simulink library "Simple_lib"  (R2018b)
settings: Solver=ode45  StartTime=0.0  StopTime=10.0  RelTol=1e-3  EnableMultiTasking=on
undefined symbols (not defined in the file or in its folder): Acceptance, beta, C, C_J, C_P, c_wall, dGain, DiscIntNeverNeededParam, Duplex, Electrical_lib, grab, h_fe, i, i3, K_T, Kman, KmanCE, mu_s, n_rev, R_arm, Simplex, systemTs, tau_0, TinIC, Ts, w_0, wallMass, Watch_lib
libraries: $bdroot x407, PlantUtilityBlockset_lib x30, peGeneralControl x22, simulink x11
(part 7 of 14)

== system Simple_lib/Electrical/Thyristor ==
  In1 : Inport
  c : Inport  Port=2
  In2 : Inport  Port=3
  1/R1 : Gain  Gain=-1
  1/R2 : Gain  Gain=-1
  Discrete-Time Integrator1 : DiscreteIntegrator  gainval=1/10/Ts  SampleTime=Ts  ICPrevOutput=DiscIntNeverNeededParam  ICPrevScaledInput=DiscIntNeverNeededParam
  Saturation : Saturate  UpperLimit=Inf  LowerLimit=0
  Simplex : $bdroot/Utility/Push  Tag=Electrical  SystemSampleTime=-1
  Simplex1 : $bdroot/Utility/Push  Tag=Electrical  SystemSampleTime=-1
  Sum : Sum  Inputs=+|+
  Sum1 : Sum  Inputs=|+-
  conductance : Product
  wires:
  Saturation/1 -> Sum1/1
  conductance/1 -> Saturation/1
  In1/1 -> Simplex/1
  Simplex/1 -> 1/R2/1
  1/R2/1 -> Sum/1
  Sum/1 -> conductance/2
  In2/1 -> Simplex1/1
  Simplex1/1 -> Sum/2
  1/R1/1 -> Simplex1/2
  Sum1/1 -> Discrete-Time Integrator1/1
  Discrete-Time Integrator1/1 -> Simplex/2, 1/R1/1, Sum1/2
  c/1 -> conductance/1

== system Simple_lib/Electrical/Tran ==
  In1 : Inport
  gain : Inport  Port=2
  Duplex : $bdroot/Utility/Output  Tag=Electrical  Level=Level  Flow=flow
  Multiply : Product
  Multiply1 : Product
  Simplex : $bdroot/Utility/Input  Tag=Electrical  Level=V  Flow=I
  Sum1 : Sum  Inputs=+
  Out1 : Outport
  wires:
  Duplex/2 -> Sum1/1
  Duplex/1 -> Out1/1
  Simplex/1 -> Multiply/1
  In1/1 -> Simplex/1
  Multiply1/1 -> Simplex/2
  Multiply/1 -> Duplex/1
  Sum1/1 -> Multiply1/2
  gain/1 -> Multiply1/1, Multiply/2

== system Simple_lib/Electrical/V ==
  C : PlantUtilityBlockset_lib/Electrical/C  C=.1
  Ground : Ground
  Out1 : Outport
  wires:
  C/1 -> Out1/1
  Ground/1 -> C/1

== system Simple_lib/Electrical/VM ==
  note: Does not need duplex
  In1 : Inport
  In2 : Inport  Port=2
  1/R2 : Gain  Gain=-1
  Sum : Sum  Inputs=+|+
  Out1 : Outport
  wires:
  In2/1 -> 1/R2/1
  Sum/1 -> Out1/1
  In1/1 -> Sum/1
  1/R2/1 -> Sum/2

== system Simple_lib/Electrical/VR ==
  In1 : Inport
  R : Inport  Port=2
  Bus Creator : BusCreator  Inputs=2
  Bus Selector : BusSelector  OutputSignals=V,R
  Inflow : $bdroot/Utility/Inflow  SystemSampleTime=-1
  Multiply : Product
  Outflow : $bdroot/Utility/Outflow  Tag=Electrical  SystemSampleTime=-1
  Sum2 : Sum  Inputs=|++
  Sum3 : Sum  Inputs=|+-
  Sum4 : Sum  Inputs=+  CollapseMode=Specified dimension  CollapseDim=2
  Out1 : Outport
  wires:
  Outflow/1 -> Out1/1
  Bus Creator/1 -> Outflow/1
  Sum3/1 -> Bus Creator/1  "V"
  Sum4/1 -> Inflow/2, Multiply/2  "I"
  Bus Selector/1 -> Sum3/1  "<V>"
  Multiply/1 -> Sum3/2
  Outflow/2 -> Sum4/1
  Inflow/1 -> Bus Selector/1
  R/1 -> Multiply/1, Sum2/2
  Sum2/1 -> Bus Creator/2  "R"
  In1/1 -> Inflow/1
  Bus Selector/2 -> Sum2/1  "<R>"

== system Simple_lib/Electrical/VS ==
  In2 : Inport
  Duplex : PlantUtilityBlockset_lib/Utility/Pull  Tag=Electrical  SystemSampleTime=-1
  Terminator : Terminator
  Out1 : Outport
  wires:
  In2/1 -> Duplex/1
  Duplex/2 -> Terminator/1
  Duplex/1 -> Out1/1

== system Simple_lib/Electrical/VStep ==
  In2 : Inport
  Duplex : PlantUtilityBlockset_lib/Utility/Pull  Tag=Electrical  SystemSampleTime=-1
  Terminator : Terminator
  Out1 : Outport
  wires:
  Duplex/1 -> Out1/1
  Duplex/2 -> Terminator/1
  In2/1 -> Duplex/1

== system Simple_lib/Electrical/Windings ==
  Eabc : Inport
  A : Inport  Port=2
  B : Inport  Port=3
  C : Inport  Port=4
  Demux : Demux  Outputs=3
  IM : Subsystem  AncestorBlock=PlantUtilityBlockset_lib/Electrical/IM  mask{R=1}
      mask prompts: R "Resistance"
      mask Display:
      | color('white')
      | plot([-1 1 1 -1 -1], [-1 -1 1 1 -1])
      | color('black')
      | plot([1.0 1.18 1.18 1.0], [0 .2 -.2 0]+.4)
      | plot([-1 -.9 -.5 0 .5 .9 1  .9  .5  0 -.5 -.9 -1],      [ 0  .5 .9 1 .9 .5 0 -.5 -.9 -1 -.9 -.5  0]);
      | text(0,0, 'A')
  IM1 : Subsystem  AncestorBlock=PlantUtilityBlockset_lib/Electrical/IM  mask{R=1}
      mask prompts: R "Resistance"
      mask Display:
      | color('white')
      | plot([-1 1 1 -1 -1], [-1 -1 1 1 -1])
      | color('black')
      | plot([1.0 1.18 1.18 1.0], [0 .2 -.2 0]+.4)
      | plot([-1 -.9 -.5 0 .5 .9 1  .9  .5  0 -.5 -.9 -1],      [ 0  .5 .9 1 .9 .5 0 -.5 -.9 -1 -.9 -.5  0]);
      | text(0,0, 'A')
  IM2 : Subsystem  AncestorBlock=PlantUtilityBlockset_lib/Electrical/IM  mask{R=1}
      mask prompts: R "Resistance"
      mask Display:
      | color('white')
      | plot([-1 1 1 -1 -1], [-1 -1 1 1 -1])
      | color('black')
      | plot([1.0 1.18 1.18 1.0], [0 .2 -.2 0]+.4)
      | plot([-1 -.9 -.5 0 .5 .9 1  .9  .5  0 -.5 -.9 -1],      [ 0  .5 .9 1 .9 .5 0 -.5 -.9 -1 -.9 -.5  0]);
      | text(0,0, 'A')
  L1 : Subsystem  AncestorBlock=PlantUtilityBlockset_lib/Electrical/L1  mask{L=1}
      mask prompts: L "Inductance"
      mask Display:
      | %color('black')
      | plot(   [    0     0.3827     0.7071     0.9239     1.0000     0.9239     0.7071     0.3827     0.0000    -0.3827    -0.7071    -0.9239    -1.0000    -0.9239    -0.7071    -0.3827    -0.0000     0.3827     0.7071     0.9239     1.0000     0.9239     0.7071     0.3827     0.0000    -0.3827    -0.7071    -0.9239    -1.0000    -0.9239    -0.7071    -0.3827    -0.0000     0.3827     0.7071     0.9239     1.0000     0.9239     0.7071     0.3827     0.0000    -0.3827    -0.7071    -0.9239    -1.0000    -0.9239    -0.7071    -0.3827    -0.0000     0.3827     0.7071     0.9239     1.0000     0.9239     0.7071     0.3827     0.0000    -0.3827    -0.7071    -0.9239    -1.0000    -0.9239    -0.7071    -0.3827    -0.0000],   -.5+[-0.0625    -0.0421    -0.0129     0.0230     0.0625     0.1020     0.1379     0.1671     0.1875     0.1984     0.2004     0.1958     0.1875     0.1792     0.1746     0.1766     0.1875     0.2079     0.2371     0.2730     0.3125     0.3520     0.3879     0.4171     0.4375     0.4484     0.4504     0.4458     0.4375     0.4292     0.4246     0.4266     0.4375     0.4579     0.4871     0.5230     0.5625     0.6020     0.6379     0.6671     0.6875     0.6984     0.7004     0.6958     0.6875     0.6792     0.6746     0.6766     0.6875     0.7079     0.7371     0.7730     0.8125     0.8520     0.8879     0.9171     0.9375     0.9484     0.9504     0.9458     0.9375     0.9292     0.9246     0.9266     0.9375])
      | color('white')
      | plot([-1 1 1 -1 -1], [-1 -1 1 1 -1])
  L2 : Subsystem  AncestorBlock=PlantUtilityBlockset_lib/Electrical/L1  mask{L=1}
      mask prompts: L "Inductance"
      mask Display:
      | %color('black')
      | plot(   [    0     0.3827     0.7071     0.9239     1.0000     0.9239     0.7071     0.3827     0.0000    -0.3827    -0.7071    -0.9239    -1.0000    -0.9239    -0.7071    -0.3827    -0.0000     0.3827     0.7071     0.9239     1.0000     0.9239     0.7071     0.3827     0.0000    -0.3827    -0.7071    -0.9239    -1.0000    -0.9239    -0.7071    -0.3827    -0.0000     0.3827     0.7071     0.9239     1.0000     0.9239     0.7071     0.3827     0.0000    -0.3827    -0.7071    -0.9239    -1.0000    -0.9239    -0.7071    -0.3827    -0.0000     0.3827     0.7071     0.9239     1.0000     0.9239     0.7071     0.3827     0.0000    -0.3827    -0.7071    -0.9239    -1.0000    -0.9239    -0.7071    -0.3827    -0.0000],   -.5+[-0.0625    -0.0421    -0.0129     0.0230     0.0625     0.1020     0.1379     0.1671     0.1875     0.1984     0.2004     0.1958     0.1875     0.1792     0.1746     0.1766     0.1875     0.2079     0.2371     0.2730     0.3125     0.3520     0.3879     0.4171     0.4375     0.4484     0.4504     0.4458     0.4375     0.4292     0.4246     0.4266     0.4375     0.4579     0.4871     0.5230     0.5625     0.6020     0.6379     0.6671     0.6875     0.6984     0.7004     0.6958     0.6875     0.6792     0.6746     0.6766     0.6875     0.7079     0.7371     0.7730     0.8125     0.8520     0.8879     0.9171     0.9375     0.9484     0.9504     0.9458     0.9375     0.9292     0.9246     0.9266     0.9375])
      | color('white')
      | plot([-1 1 1 -1 -1], [-1 -1 1 1 -1])
  L3 : Subsystem  AncestorBlock=PlantUtilityBlockset_lib/Electrical/L1  mask{L=1}
      mask prompts: L "Inductance"
      mask Display:
      | %color('black')
      | plot(   [    0     0.3827     0.7071     0.9239     1.0000     0.9239     0.7071     0.3827     0.0000    -0.3827    -0.7071    -0.9239    -1.0000    -0.9239    -0.7071    -0.3827    -0.0000     0.3827     0.7071     0.9239     1.0000     0.9239     0.7071     0.3827     0.0000    -0.3827    -0.7071    -0.9239    -1.0000    -0.9239    -0.7071    -0.3827    -0.0000     0.3827     0.7071     0.9239     1.0000     0.9239     0.7071     0.3827     0.0000    -0.3827    -0.7071    -0.9239    -1.0000    -0.9239    -0.7071    -0.3827    -0.0000     0.3827     0.7071     0.9239     1.0000     0.9239     0.7071     0.3827     0.0000    -0.3827    -0.7071    -0.9239    -1.0000    -0.9239    -0.7071    -0.3827    -0.0000],   -.5+[-0.0625    -0.0421    -0.0129     0.0230     0.0625     0.1020     0.1379     0.1671     0.1875     0.1984     0.2004     0.1958     0.1875     0.1792     0.1746     0.1766     0.1875     0.2079     0.2371     0.2730     0.3125     0.3520     0.3879     0.4171     0.4375     0.4484     0.4504     0.4458     0.4375     0.4292     0.4246     0.4266     0.4375     0.4579     0.4871     0.5230     0.5625     0.6020     0.6379     0.6671     0.6875     0.6984     0.7004     0.6958     0.6875     0.6792     0.6746     0.6766     0.6875     0.7079     0.7371     0.7730     0.8125     0.8520     0.8879     0.9171     0.9375     0.9484     0.9504     0.9458     0.9375     0.9292     0.9246     0.9266     0.9375])
      | color('white')
      | plot([-1 1 1 -1 -1], [-1 -1 1 1 -1])
  Mux : Mux  Inputs=3
  R : Subsystem  AncestorBlock=PlantUtilityBlockset_lib/Electrical/R  mask{R=1}
      mask prompts: R "Resistance"
      mask Display:
      | color('white')
      | plot([-1 1 1 -1 -1], [-1 -1 1 1 -1])
      | color('black')
      | plot([1.0 1.18 1.18 1.0], [0 .2 -.2 0])
      | plot([-8:8]/8, [0 1 0 -1 0 1 0 -1 0 1 0 -1 0 1 0 -1 0])
  R1 : Subsystem  AncestorBlock=PlantUtilityBlockset_lib/Electrical/R  mask{R=1}
      mask prompts: R "Resistance"
      mask Display:
      | color('white')
      | plot([-1 1 1 -1 -1], [-1 -1 1 1 -1])
      | color('black')
      | plot([1.0 1.18 1.18 1.0], [0 .2 -.2 0])
      | plot([-8:8]/8, [0 1 0 -1 0 1 0 -1 0 1 0 -1 0 1 0 -1 0])
  R2 : Subsystem  AncestorBlock=PlantUtilityBlockset_lib/Electrical/R  mask{R=1}
      mask prompts: R "Resistance"
      mask Display:
      | color('white')
      | plot([-1 1 1 -1 -1], [-1 -1 1 1 -1])
      | color('black')
      | plot([1.0 1.18 1.18 1.0], [0 .2 -.2 0])
      | plot([-8:8]/8, [0 1 0 -1 0 1 0 -1 0 1 0 -1 0 1 0 -1 0])
  Terminator : Terminator
  Terminator1 : Terminator
  Terminator2 : Terminator
  Va : Subsystem  Tag=Electrical  AncestorBlock=PlantUtilityBlockset_lib/Utility/Pull  InitFcn=initDuplex
      mask Display:
      | color('white')
      | plot([0 3], [2 2])
      | plot([0 3], [-2 -2])
      | color('black')
      | 
      | plot([0 1 1], [0 0 0.4])
      | plot([1 1 3], [0.6 1 1])
      | plot([1 3 2 1 0 2], [0.6 0.6 0.4 0.6 0.4 0.4])
      | patch([0 2 1],[0.4 0.4 0.6],[0,0,0])
      | plot([3 2 2], [1 1 0.6])
      | plot([2 2 3], [0.4 -1 -1])
  Vb : Subsystem  Tag=Electrical  AncestorBlock=PlantUtilityBlockset_lib/Utility/Pull  InitFcn=initDuplex
      mask Display:
      | color('white')
      | plot([0 3], [2 2])
      | plot([0 3], [-2 -2])
      | color('black')
      | 
      | plot([0 1 1], [0 0 0.4])
      | plot([1 1 3], [0.6 1 1])
      | plot([1 3 2 1 0 2], [0.6 0.6 0.4 0.6 0.4 0.4])
      | patch([0 2 1],[0.4 0.4 0.6],[0,0,0])
      | plot([3 2 2], [1 1 0.6])
      | plot([2 2 3], [0.4 -1 -1])
  Vc : Subsystem  Tag=Electrical  AncestorBlock=PlantUtilityBlockset_lib/Utility/Pull  InitFcn=initDuplex
      mask Display:
      | color('white')
      | plot([0 3], [2 2])
      | plot([0 3], [-2 -2])
      | color('black')
      | 
      | plot([0 1 1], [0 0 0.4])
      | plot([1 1 3], [0.6 1 1])
      | plot([1 3 2 1 0 2], [0.6 0.6 0.4 0.6 0.4 0.4])
      | patch([0 2 1],[0.4 0.4 0.6],[0,0,0])
      | plot([3 2 2], [1 1 0.6])
      | plot([2 2 3], [0.4 -1 -1])
  i : Outport  InitialOutput=0
  wires:
  Mux/1 -> i/1
  Demux/3 -> Vc/1(InPot)
  Demux/2 -> Vb/1(InPot)
  Demux/1 -> Va/1(InPot)
  Eabc/1 -> Demux/1
  Va/1(OutPot) -> R/1(In1)
  R/1(Out1) -> IM/1(In1)
  R1/1(Out1) -> IM1/1(In1)
  C/1 -> L3/2(In2)
  B/1 -> L2/2(In2)
  A/1 -> L1/2(In2)
  Vb/1(OutPot) -> R1/1(In1)
  Vc/1(OutPot) -> R2/1(In1)
  IM/1(Out1) -> L1/1(In1)
  IM1/1(Out1) -> L2/1(In1)
  R2/1(Out1) -> IM2/1(In1)
  IM2/1(Out1) -> L3/1(In1)
  IM2/2(Out2) -> Mux/3
  IM1/2(Out2) -> Mux/2
  IM/2(Out2) -> Mux/1
  Vc/2(OutFlow) -> Terminator2/1
  Vb/2(OutFlow) -> Terminator1/1
  Va/2(OutFlow) -> Terminator/1

== system Simple_lib/Electrical/h_params_old ==
  In1 : Inport
  Duplex : $bdroot/Utility/Output  Tag=Electrical  Level=Level  Flow=flow
  Simplex : $bdroot/Utility/Input  Tag=Electrical  Level=V  Flow=I
  Sum1 : Sum  Inputs=+
  h_fe : Gain  Gain=100
  h_re : Gain  Gain=1e-6
  Out1 : Outport
  wires:
  Duplex/2 -> Sum1/1
  Duplex/1 -> Out1/1
  Simplex/1 -> h_re/1
  In1/1 -> Simplex/1
  h_fe/1 -> Simplex/2
  h_re/1 -> Duplex/1
  Sum1/1 -> h_fe/1

== system Simple_lib/Electrical/meter ==
  In1 : Inport
  Duplex : $bdroot/Utility/Output  Tag=Electrical  Level=Level  Flow=flow
  Multiply : Product
  Power : Scope
  Simplex : $bdroot/Utility/Input  Tag=Electrical  Level=V  Flow=I
  Sum1 : Sum  Inputs=+
  flow : Scope
  level : Scope
  Out1 : Outport
  wires:
  Simplex/1 -> level/1, Duplex/1, Multiply/1
  Duplex/1 -> Out1/1
  Sum1/1 -> flow/1, Multiply/2, Simplex/2
  In1/1 -> Simplex/1
  Duplex/2 -> Sum1/1
  Multiply/1 -> Power/1

== system Simple_lib/Electronics/Ammeter ==
  Bus Selector : BusSelector  OutputSignals=I
  Constant : Constant  Value=0
  _out : $bdroot/Electronics/_out  Tag=Electrical  Level=V  Flow=I
  Sys : Outport
  I : Outport  Port=2
  wires:
  _out/1 -> Sys/1
  _out/2 -> Bus Selector/1
  Constant/1 -> _out/1
  Bus Selector/1 -> I/1  "<I>"

== system Simple_lib/Electronics/BiGain ==
  w : Inport
  Bus Creator1 : BusCreator  Inputs=2
  Bus Selector : BusSelector  OutputSignals=I,C
  Ground : Ground
  Terminator : Terminator
  _in1 : $bdroot/Electronics/_in  Level=V  Flow=I
  _out : Subsystem  Tag=Electrical  AncestorBlock=Simple_lib/Electronics/_out  mask{Level=V, Flow=I}
      mask prompts: Level "Level variable name:"; Flow "Flow variable name:"
      mask init:
      | init_out
      mask Display:
      | % This is a new mask on top of the base mask.
      | % Use "View base mask" link below to see the base mask.
      | % Icon for flow out
      | %% Complex icon
      | %plot([0 1 1], [0 0 0.4])
      | %plot([1 1 3], [0.6 1 1])
      | %plot([1 3 2 1 0 2], [0.6 0.6 0.4 0.6 0.4 0.4])
      | %patch([0 2 1],[0.4 0.4 0.6])
      | %plot([3 2 2], [1 1 0.6])
      | %plot([2.2 2.2], [1 0.6])
      | %plot([1.8 1.8], [1 0.6])
      | %plot([1.6 2.4], [0 0])
      | %plot([2 2], [0.1 -0.1])
      | %plot([2 2], [0.4 0.2])
      | %plot([2 2 3], [-0.2 -1 -1])
      | 
      | %color('white')
      | %plot([0 3], [2 2])
      | %plot([0 3], [-2 -2])
      | 
      | %% Bolder icon
      | plot([-1 0 1], [0 -1 0])
      | %patch([-1 1 0 -1], [1 1 2 1]*1-1)
      | patch([-1 -.2 -.2], [0 0 1])
      | patch([1 .2 .2], [0 0 1])
      | %patch( [-0.1 0.1 0.1 -0.1], [0 0 1 1], [1 1 1])
      | plot(0.2*[-1 1],-0.3*[1  1]+0*1.5)
      | plot([0 0],[-0.15 -0.45]+0*1.5)
      | 
      | 
      | color('white')
      | plot( [-1 1], [2 2])
      | plot( [-1 1], -[2 2])
  k_flow1 : Gain  Gain=k_flow
  k_pot : Gain  Gain=k_level
  V : Outport
  wires:
  _out/1(out) -> V/1
  Ground/1 -> Bus Creator1/2  "J"
  Bus Selector/2 -> Terminator/1  "<C>"
  w/1 -> _in1/1
  _out/2(backs) -> Bus Selector/1
  k_pot/1 -> _out/1(in)
  Bus Creator1/1 -> _in1/2
  k_flow1/1 -> Bus Creator1/1  "tau"
  _in1/1 -> k_pot/1
  Bus Selector/1 -> k_flow1/1  "<I>"

== system Simple_lib/Electronics/C ==
  In1 : Inport
  Capacitance : $bdroot/Electronics/Capacitance  C=C
      settings: AttributesFormatString=%<C> F
  Ground : Ground
  M : $bdroot/Electronics/M1  SystemSampleTime=-1
  Sum : Sum  Inputs=|++
  extra : $bdroot/Electronics/TP  V_0=0.0  slew_rate=100.0  conserved_quantity_name=Q  energy_name=E
  Out1 : Outport
  wires:
  Sum/1 -> M/1
  In1/1 -> Sum/1
  extra/1 -> Capacitance/1, Sum/2
  M/1 -> Out1/1
  Ground/1 -> extra/1

== system Simple_lib/Electronics/C1 ==
  pos : Inport
  neg : Inport  Port=2
  1/R3 : Gain  Gain=-1
  Bus Creator : BusCreator  Inputs=3
  Bus Creator1 : BusCreator  Inputs=3
  Constant1 : Constant  Value=C
  Discrete-Time Integrator : DiscreteIntegrator  SampleTime=-1  ICPrevOutput=DiscIntNeverNeededParam  ICPrevScaledInput=DiscIntNeverNeededParam
  Gain1 : Gain  Gain=C
  Gain2 : Gain  Gain=1/C
  Ground : Ground
  Sum2 : Sum  Inputs=+--
  Weighted Sample Time : SampleTimeMath  TsampMathOp=/  weightValue=2
  _neg : $bdroot/Electronics/_in  Level=V  Flow=I
  _pos : $bdroot/Electronics/_in  Level=V  Flow=I
  wires:
  Gain2/1 -> Discrete-Time Integrator/1  "I"
  Discrete-Time Integrator/1 -> Sum2/2
  Gain1/1 -> Gain2/1, Bus Creator/1, 1/R3/1  "I"
  Weighted Sample Time/1 -> Gain1/1
  neg/1 -> _neg/1
  pos/1 -> _pos/1
  _pos/1 -> Sum2/1
  Bus Creator/1 -> _pos/2
  Bus Creator1/1 -> _neg/2
  _neg/1 -> Sum2/3
  Sum2/1 -> Weighted Sample Time/1
  1/R3/1 -> Bus Creator1/3  "I"
  Ground/1 -> Bus Creator/2, Bus Creator1/2  "G"
  Constant1/1 -> Bus Creator1/1, Bus Creator/3  "C"

== system Simple_lib/Electronics/Capacitance ==
  In2 : Inport
  Bus Creator : BusCreator  Inputs=3
  Constant : Constant  Value=C
  Ground : Ground
  Ground1 : Ground
  Terminator : Terminator
  _at : $bdroot/Electronics/_in  Level=V  Flow=I
  wires:
  Bus Creator/1 -> _at/2
  Ground/1 -> Bus Creator/2  "I"
  _at/1 -> Terminator/1
  In2/1 -> _at/1
  Constant/1 -> Bus Creator/3  "C"
  Ground1/1 -> Bus Creator/1  "G"

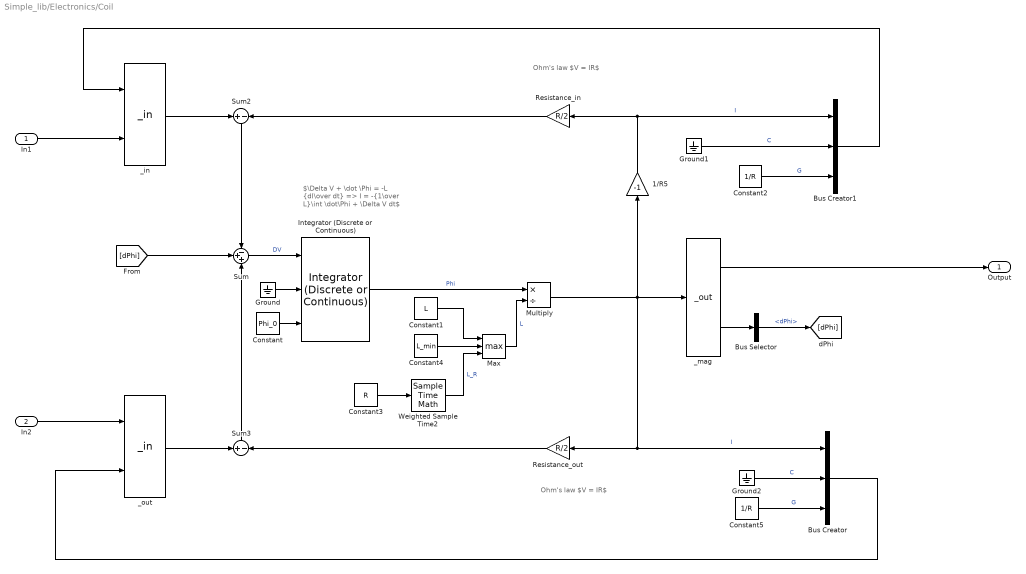
== system Simple_lib/Electronics/Coil ==
  note: Ohm's law $V = IR$
  note: $\Delta V + \dot \Phi = -L {dI\over dt} => I = -{1\over L}\int \dot\Phi + \Delta V dt$
  note: Ohm's law $V = IR$
  In1 : Inport
  In2 : Inport  Port=2
  1/R5 : Gain  Gain=-1
  Bus Creator : BusCreator  Inputs=3
  Bus Creator1 : BusCreator  Inputs=3
  Bus Selector : BusSelector  OutputSignals=dPhi
  Constant : Constant  Value=Phi_0
  Constant1 : Constant  Value=L
  Constant2 : Constant  Value=1/R
  Constant3 : Constant  Value=R
  Constant4 : Constant  Value=L_min
  Constant5 : Constant  Value=1/R
  Ground : Ground
  Ground1 : Ground
  Ground2 : Ground
  Integrator (Discrete or Continuous) : peGeneralControl/Integrator (Discrete or Continuous)  LabelModeActiveChoice=Discrete  ExternalReset=level  LimitType=Anti-windup  B=inf  A=-inf  Ts=systemTs
  Max : MinMax  Function=max  Inputs=3
  Multiply : Product  Inputs=*/
  Resistance_in : Gain  Gain=R/2
  Resistance_out : Gain  Gain=R/2
  Sum : Sum  Inputs=-++
  Sum2 : Sum  Inputs=+|-
  Sum3 : Sum  Inputs=+|-
  Weighted Sample Time2 : SampleTimeMath  TsampMathOp=*  weightValue=1
  _in : $bdroot/Electronics/_in  Level=V  Flow=I
      mask init:
      | initInput
      mask Display:
      | % This is a new mask on top of the base mask.
      | % Use "View base mask" link below to see the base mask.
      | %% Icon for flow in
      | % Signally design
      | %plot([0 2 2 3], [1 1 0 0])
      | %plot([1 3 2 1 0 2], [0.6 0.6 0.4 0.6 0.4 0.4])
      | %patch([1 3 2],[0.6 0.6 0.4])
      | %plot([0 1 1], [1 1 0.6])
      | %plot([1 1 0], [0.4 -1 -1])
      | 
      | %color('white')
      | %plot([0 3], [2 2])
      | %plot([0 3], [-2 -2])
      | 
      | %% Bolder design
      | %patch( [0 1 -1], [0 1 1])
      | patch( [-0.1 -0.1 -1], [0.95 0 0.95])
      | patch( [0.1 0.1 1], [1 0 1])
      | plot( [0.1 1 -1 -0.1], [0 -2 -2 0]*0.5)
      | %patch( [-0.1 0.1 0.1 -0.1], [0 0 1 1], [1 1 1])
      | %patch( [-1 0.1 0.1 -1], [1 1 0.95 0.95], [1 1 1])
      | 
      | %% Size the box
      | color('white')
      | plot( [-1 1], [2 2])
      | plot( [-1 1], -[2 2])
  _mag : $bdroot/Magnetic/_out  Tag=Electrical  Level=v  Flow=F
  _out : $bdroot/Electronics/_in  Level=V  Flow=I
      mask init:
      | initInput
      mask Display:
      | % This is a new mask on top of the base mask.
      | % Use "View base mask" link below to see the base mask.
      | %% Icon for flow in
      | % Signally design
      | %plot([0 2 2 3], [1 1 0 0])
      | %plot([1 3 2 1 0 2], [0.6 0.6 0.4 0.6 0.4 0.4])
      | %patch([1 3 2],[0.6 0.6 0.4])
      | %plot([0 1 1], [1 1 0.6])
      | %plot([1 1 0], [0.4 -1 -1])
      | 
      | %color('white')
      | %plot([0 3], [2 2])
      | %plot([0 3], [-2 -2])
      | 
      | %% Bolder design
      | %patch( [0 1 -1], [0 1 1])
      | patch( [-0.1 -0.1 -1], [0.95 0 0.95])
      | patch( [0.1 0.1 1], [1 0 1])
      | plot( [0.1 1 -1 -0.1], [0 -2 -2 0]*0.5)
      | %patch( [-0.1 0.1 0.1 -0.1], [0 0 1 1], [1 1 1])
      | %patch( [-1 0.1 0.1 -1], [1 1 0.95 0.95], [1 1 1])
      | 
      | %% Size the box
      | color('white')
      | plot( [-1 1], [2 2])
      | plot( [-1 1], -[2 2])
  Output : Outport
  wires:
  Constant5/1 -> Bus Creator/3  "G"
  Ground2/1 -> Bus Creator/2  "C"
  Bus Selector/1 -> [dPhi]  "<dPhi>"
  Ground/1 -> Integrator (Discrete or Continuous)/2
  Constant/1 -> Integrator (Discrete or Continuous)/3
  Ground1/1 -> Bus Creator1/2  "C"
  Constant2/1 -> Bus Creator1/3  "G"
  Sum3/1 -> Sum/3
  Sum2/1 -> Sum/1
  In1/1 -> _in/1
  1/R5/1 -> Bus Creator1/1, Resistance_in/1  "I"
  Resistance_in/1 -> Sum2/2
  _in/1 -> Sum2/1
  Integrator (Discrete or Continuous)/1 -> Multiply/1  "Phi"
  In2/1 -> _out/1
  _out/1 -> Sum3/1
  Resistance_out/1 -> Sum3/2
  Bus Creator/1 -> _out/2
  Bus Creator1/1 -> _in/2
  Multiply/1 -> 1/R5/1, _mag/1, Resistance_out/1, Bus Creator/1  "I"
  Max/1 -> Multiply/2  "L"
  Sum/1 -> Integrator (Discrete or Continuous)/1  "DV"
  Constant1/1 -> Max/1
  Constant3/1 -> Weighted Sample Time2/1
  Weighted Sample Time2/1 -> Max/3  "L_R"
  _mag/2 -> Bus Selector/1
  _mag/1 -> Output/1
  [dPhi] -> Sum/2
  Constant4/1 -> Max/2

== system Simple_lib/Electronics/Csav ==
  In1 : Inport
  Bus Selector : BusSelector  OutputSignals=I
  Constant : Constant  Value=Q_0
  Gain : Gain  Gain=1/C
  Ground : Ground
  Integrator (Discrete or Continuous) : peGeneralControl/Integrator (Discrete or Continuous)  LabelModeActiveChoice=Discrete  ExternalReset=level  LimitType=Anti-windup  B=inf  A=-inf  Ts=-1
  Sum : Sum  Inputs=|+-
  _in : $bdroot/Electronics/_in  Level=V  Flow=I
      mask init:
      | initInput
      mask Display:
      | % This is a new mask on top of the base mask.
      | % Use "View base mask" link below to see the base mask.
      | %% Icon for flow in
      | % Signally design
      | %plot([0 2 2 3], [1 1 0 0])
      | %plot([1 3 2 1 0 2], [0.6 0.6 0.4 0.6 0.4 0.4])
      | %patch([1 3 2],[0.6 0.6 0.4])
      | %plot([0 1 1], [1 1 0.6])
      | %plot([1 1 0], [0.4 -1 -1])
      | 
      | %color('white')
      | %plot([0 3], [2 2])
      | %plot([0 3], [-2 -2])
      | 
      | %% Bolder design
      | %patch( [0 1 -1], [0 1 1])
      | patch( [-0.1 -0.1 -1], [0.95 0 0.95])
      | patch( [0.1 0.1 1], [1 0 1])
      | plot( [0.1 1 -1 -0.1], [0 -2 -2 0]*0.5)
      | %patch( [-0.1 0.1 0.1 -0.1], [0 0 1 1], [1 1 1])
      | %patch( [-1 0.1 0.1 -1], [1 1 0.95 0.95], [1 1 1])
      | 
      | %% Size the box
      | color('white')
      | plot( [-1 1], [2 2])
      | plot( [-1 1], -[2 2])
  _out : $bdroot/Electronics/_out  Tag=Electrical  Level=V  Flow=I
  Out1 : Outport
  wires:
  Gain/1 -> Sum/2
  Ground/1 -> Integrator (Discrete or Continuous)/2
  Constant/1 -> Integrator (Discrete or Continuous)/3
  Bus Selector/1 -> Integrator (Discrete or Continuous)/1  "<I>"
  _out/2 -> _in/2, Bus Selector/1
  Sum/1 -> _out/1
  _in/1 -> Sum/1
  _out/1 -> Out1/1
  In1/1 -> _in/1
  Integrator (Discrete or Continuous)/1 -> Gain/1

== system Simple_lib/Electronics/Csav2 ==
  In1 : Inport
  Bus Selector : BusSelector  OutputSignals=I
  Constant : Constant  Value=Q_0
  Gain : Gain  Gain=1/C
  Ground : Ground
  Integrator (Discrete or Continuous) : peGeneralControl/Integrator (Discrete or Continuous)  LabelModeActiveChoice=Discrete  ExternalReset=level  LimitType=Anti-windup  B=inf  A=-inf  Ts=-1
  Sum : Sum  Inputs=|+-
  _in : $bdroot/Electronics/_in  Level=V  Flow=I
      mask init:
      | initInput
      mask Display:
      | % This is a new mask on top of the base mask.
      | % Use "View base mask" link below to see the base mask.
      | %% Icon for flow in
      | % Signally design
      | %plot([0 2 2 3], [1 1 0 0])
      | %plot([1 3 2 1 0 2], [0.6 0.6 0.4 0.6 0.4 0.4])
      | %patch([1 3 2],[0.6 0.6 0.4])
      | %plot([0 1 1], [1 1 0.6])
      | %plot([1 1 0], [0.4 -1 -1])
      | 
      | %color('white')
      | %plot([0 3], [2 2])
      | %plot([0 3], [-2 -2])
      | 
      | %% Bolder design
      | %patch( [0 1 -1], [0 1 1])
      | patch( [-0.1 -0.1 -1], [0.95 0 0.95])
      | patch( [0.1 0.1 1], [1 0 1])
      | plot( [0.1 1 -1 -0.1], [0 -2 -2 0]*0.5)
      | %patch( [-0.1 0.1 0.1 -0.1], [0 0 1 1], [1 1 1])
      | %patch( [-1 0.1 0.1 -1], [1 1 0.95 0.95], [1 1 1])
      | 
      | %% Size the box
      | color('white')
      | plot( [-1 1], [2 2])
      | plot( [-1 1], -[2 2])
  _out : $bdroot/Electronics/_out  Tag=Electrical  Level=V  Flow=I
  Out1 : Outport
  wires:
  Integrator (Discrete or Continuous)/1 -> Gain/1
  In1/1 -> _in/1
  _out/1 -> Out1/1
  _in/1 -> Sum/1
  Sum/1 -> _out/1
  _out/2 -> Bus Selector/1, _in/2
  Bus Selector/1 -> Integrator (Discrete or Continuous)/1  "<I>"
  Constant/1 -> Integrator (Discrete or Continuous)/3
  Ground/1 -> Integrator (Discrete or Continuous)/2
  Gain/1 -> Sum/2

== system Simple_lib/Electronics/CurrentSource ==
  I : Inport
  Sys : Inport  Port=2
  Terminator : Terminator
  _in : $bdroot/Electronics/_in  Level=V  Flow=I
  wires:
  I/1 -> _in/2
  Sys/1 -> _in/1
  _in/1 -> Terminator/1

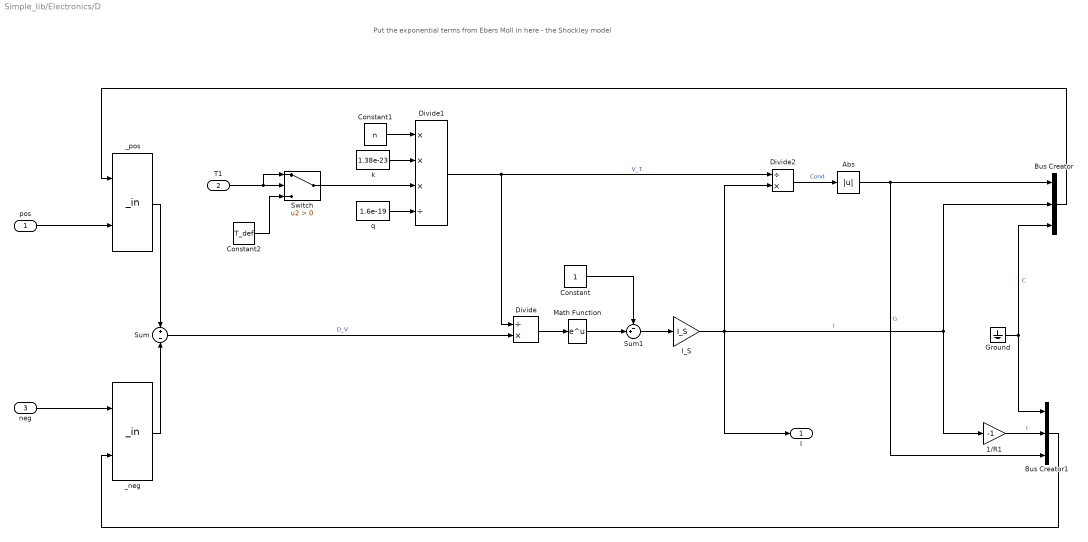
== system Simple_lib/Electronics/D ==
  note: Put the exponential terms from Ebers Moll in here - the Shockley model
  pos : Inport
  T1 : Inport  Port=2
  neg : Inport  Port=3
  1/R1 : Gain  Gain=-1
  Abs : Abs
  Bus Creator : BusCreator  Inputs=3
  Bus Creator1 : BusCreator  Inputs=3
  Constant : Constant
  Constant1 : Constant  Value=n
  Constant2 : Constant  Value=T_def
  Divide : Product  Inputs=/*
  Divide1 : Product  Inputs=***/
  Divide2 : Product  Inputs=/*
  Ground : Ground
  I_S : Gain  Gain=I_S
  Math Function : Math  SaturateOnIntegerOverflow=on
  Sum : Sum  Inputs=+|-
  Sum1 : Sum  Inputs=-+|
  Switch : Switch  Criteria=u2 > Threshold
  _neg : $bdroot/Electronics/_in  Level=V  Flow=I
      mask init:
      | initInput
      mask Display:
      | % This is a new mask on top of the base mask.
      | % Use "View base mask" link below to see the base mask.
      | %% Icon for flow in
      | % Signally design
      | %plot([0 2 2 3], [1 1 0 0])
      | %plot([1 3 2 1 0 2], [0.6 0.6 0.4 0.6 0.4 0.4])
      | %patch([1 3 2],[0.6 0.6 0.4])
      | %plot([0 1 1], [1 1 0.6])
      | %plot([1 1 0], [0.4 -1 -1])
      | 
      | %color('white')
      | %plot([0 3], [2 2])
      | %plot([0 3], [-2 -2])
      | 
      | %% Bolder design
      | %patch( [0 1 -1], [0 1 1])
      | patch( [-0.1 -0.1 -1], [0.95 0 0.95])
      | patch( [0.1 0.1 1], [1 0 1])
      | plot( [0.1 1 -1 -0.1], [0 -2 -2 0]*0.5)
      | %patch( [-0.1 0.1 0.1 -0.1], [0 0 1 1], [1 1 1])
      | %patch( [-1 0.1 0.1 -1], [1 1 0.95 0.95], [1 1 1])
      | 
      | %% Size the box
      | color('white')
      | plot( [-1 1], [2 2])
      | plot( [-1 1], -[2 2])
  _pos : $bdroot/Electronics/_in  Level=V  Flow=I
      mask init:
      | initInput
      mask Display:
      | % This is a new mask on top of the base mask.
      | % Use "View base mask" link below to see the base mask.
      | %% Icon for flow in
      | % Signally design
      | %plot([0 2 2 3], [1 1 0 0])
      | %plot([1 3 2 1 0 2], [0.6 0.6 0.4 0.6 0.4 0.4])
      | %patch([1 3 2],[0.6 0.6 0.4])
      | %plot([0 1 1], [1 1 0.6])
      | %plot([1 1 0], [0.4 -1 -1])
      | 
      | %color('white')
      | %plot([0 3], [2 2])
      | %plot([0 3], [-2 -2])
      | 
      | %% Bolder design
      | %patch( [0 1 -1], [0 1 1])
      | patch( [-0.1 -0.1 -1], [0.95 0 0.95])
      | patch( [0.1 0.1 1], [1 0 1])
      | plot( [0.1 1 -1 -0.1], [0 -2 -2 0]*0.5)
      | %patch( [-0.1 0.1 0.1 -0.1], [0 0 1 1], [1 1 1])
      | %patch( [-1 0.1 0.1 -1], [1 1 0.95 0.95], [1 1 1])
      | 
      | %% Size the box
      | color('white')
      | plot( [-1 1], [2 2])
      | plot( [-1 1], -[2 2])
  k : Constant  Value=1.38e-23
  q : Constant  Value=1.6e-19
  I : Outport
  wires:
  T1/1 -> Switch/2, Switch/1
  Constant2/1 -> Switch/3
  Constant1/1 -> Divide1/1
  1/R1/1 -> Bus Creator1/2  "I"
  Bus Creator/1 -> _pos/2
  Abs/1 -> Bus Creator/1, Bus Creator1/3  "G"
  k/1 -> Divide1/2
  Divide1/1 -> Divide2/1, Divide/1  "V_T"
  q/1 -> Divide1/4
  Switch/1 -> Divide1/3
  Divide/1 -> Math Function/1
  pos/1 -> _pos/1
  _pos/1 -> Sum/1
  Sum/1 -> Divide/2  "D_V"
  neg/1 -> _neg/1
  Sum1/1 -> I_S/1
  Constant/1 -> Sum1/1
  Math Function/1 -> Sum1/2
  _neg/1 -> Sum/2
  I_S/1 -> I/1, 1/R1/1, Bus Creator/2, Divide2/2  "I"
  Divide2/1 -> Abs/1  "Cond"
  Bus Creator1/1 -> _neg/2
  Ground/1 -> Bus Creator/3, Bus Creator1/1  "C"

== system Simple_lib/Electronics/DC Motor ==
  V_1 : Inport
  V_2 : Inport  Port=2
  BiGain : $bdroot/Electrical/BiGain  k_level=k_flow  k_flow=k_flow
      settings: AttributesFormatString="%<k_flow>   %<k_level>"
  Inertia : $bdroot/Rotational/Inertia  I=J_mot
      settings: AttributesFormatString=%<I> kgm^2
  Lump : $bdroot/Rotational/Lump  w_0=0
      settings: AttributesFormatString=%<w_0> rad/s
  R : $bdroot/Electronics/R  R=R_arm
      settings: AttributesFormatString=%<R> Ohms
  Sum : Sum  Inputs=-+|
  w : Outport
  wires:
  BiGain/1 -> Sum/1  "V"
  Sum/1 -> R/1
  V_2/1 -> R/2  "V"
  V_1/1 -> Sum/2  "V_1"
  Lump/1 -> BiGain/1, w/1, Inertia/1

== system Simple_lib/Electronics/D_1 ==
  in : Inport
  out : Inport  Port=2
  Constant : Constant  Value=g_on
  Constant1 : Constant  Value=g_off
  E : $bdroot/Electronics/E  Vbatt=-V_drop
      settings: AttributesFormatString=EMF: %<Vbatt> V
  Sum : Sum  Inputs=+|-
  Switch : Switch  Criteria=u2 > Threshold
  VR : $bdroot/Electronics/VR  SystemSampleTime=-1
  I : Outport
  wires:
  out/1 -> E/1
  Switch/1 -> VR/2
  Sum/1 -> Switch/2
  Constant/1 -> Switch/1
  Constant1/1 -> Switch/3
  VR/1 -> I/1
  in/1 -> Sum/1, VR/1
  E/1 -> Sum/2, VR/3

== system Simple_lib/Electronics/D_RR ==
  in : Inport
  out : Inport  Port=2
  1/R1 : Gain  Gain=-1
  Abs : Abs
  Bus Creator : BusCreator  Inputs=3
  Bus Creator1 : BusCreator  Inputs=3
  CondD : Gain  Gain=g
  Constant : Constant
  Constant1 : Constant  Value=V_drop
  Divide : Product  Inputs=/*
  Ground : Ground
  I_S : Gain  Gain=1/2
  Multiply : Product
  Saturation1 : Saturate  UpperLimit=inf  LowerLimit=0
  Sum : Sum  Inputs=+--
  Sum1 : Sum  Inputs=++|
  Tanh : Trigonometry  Operator=tanh
  _in : $bdroot/Electronics/_in  Level=V  Flow=I
      mask init:
      | initInput
      mask Display:
      | % This is a new mask on top of the base mask.
      | % Use "View base mask" link below to see the base mask.
      | %% Icon for flow in
      | % Signally design
      | %plot([0 2 2 3], [1 1 0 0])
      | %plot([1 3 2 1 0 2], [0.6 0.6 0.4 0.6 0.4 0.4])
      | %patch([1 3 2],[0.6 0.6 0.4])
      | %plot([0 1 1], [1 1 0.6])
      | %plot([1 1 0], [0.4 -1 -1])
      | 
      | %color('white')
      | %plot([0 3], [2 2])
      | %plot([0 3], [-2 -2])
      | 
      | %% Bolder design
      | %patch( [0 1 -1], [0 1 1])
      | patch( [-0.1 -0.1 -1], [0.95 0 0.95])
      | patch( [0.1 0.1 1], [1 0 1])
      | plot( [0.1 1 -1 -0.1], [0 -2 -2 0]*0.5)
      | %patch( [-0.1 0.1 0.1 -0.1], [0 0 1 1], [1 1 1])
      | %patch( [-1 0.1 0.1 -1], [1 1 0.95 0.95], [1 1 1])
      | 
      | %% Size the box
      | color('white')
      | plot( [-1 1], [2 2])
      | plot( [-1 1], -[2 2])
  _out : $bdroot/Electronics/_in  Level=V  Flow=I
      mask init:
      | initInput
      mask Display:
      | % This is a new mask on top of the base mask.
      | % Use "View base mask" link below to see the base mask.
      | %% Icon for flow in
      | % Signally design
      | %plot([0 2 2 3], [1 1 0 0])
      | %plot([1 3 2 1 0 2], [0.6 0.6 0.4 0.6 0.4 0.4])
      | %patch([1 3 2],[0.6 0.6 0.4])
      | %plot([0 1 1], [1 1 0.6])
      | %plot([1 1 0], [0.4 -1 -1])
      | 
      | %color('white')
      | %plot([0 3], [2 2])
      | %plot([0 3], [-2 -2])
      | 
      | %% Bolder design
      | %patch( [0 1 -1], [0 1 1])
      | patch( [-0.1 -0.1 -1], [0.95 0 0.95])
      | patch( [0.1 0.1 1], [1 0 1])
      | plot( [0.1 1 -1 -0.1], [0 -2 -2 0]*0.5)
      | %patch( [-0.1 0.1 0.1 -0.1], [0 0 1 1], [1 1 1])
      | %patch( [-1 0.1 0.1 -1], [1 1 0.95 0.95], [1 1 1])
      | 
      | %% Size the box
      | color('white')
      | plot( [-1 1], [2 2])
      | plot( [-1 1], -[2 2])
  I : Outport
  wires:
  1/R1/1 -> Bus Creator1/2  "I"
  Bus Creator/1 -> _in/2
  Divide/1 -> Tanh/1
  in/1 -> _in/1
  _in/1 -> Sum/1
  Sum/1 -> Divide/2, Multiply/2  "D_V"
  out/1 -> _out/1
  Sum1/1 -> I_S/1
  Constant/1 -> Sum1/1
  Tanh/1 -> Sum1/2
  _out/1 -> Sum/3
  I_S/1 -> CondD/1  "I"
  CondD/1 -> Abs/1, Multiply/1  "Cond"
  Bus Creator1/1 -> _out/2
  Multiply/1 -> Saturation1/1
  Constant1/1 -> Divide/1, Sum/2
  Saturation1/1 -> I/1, 1/R1/1, Bus Creator/2  "I"
  Abs/1 -> Bus Creator1/1, Bus Creator/1  "G"
  Ground/1 -> Bus Creator1/3, Bus Creator/3  "C"

== system Simple_lib/Electronics/E ==
  in : Inport
  Constant : Constant  Value=Vbatt
  Sum : Sum  Inputs=|++
  _at : $bdroot/Electronics/_out  Tag=Electrical  Level=V  Flow=I
  _thru : $bdroot/Electronics/_in  Level=V  Flow=I
  out : Outport
  wires:
  _at/1 -> out/1
  _thru/1 -> Sum/1
  Constant/1 -> Sum/2
  Sum/1 -> _at/1
  in/1 -> _thru/1
  _at/2 -> _thru/2

== system Simple_lib/Electronics/Earth ==
  Constant : Constant  Value=0
  Terminator : Terminator
  _out : $bdroot/Electronics/_out  Tag=Electrical  Level=V  Flow=I
  Output : Outport
  wires:
  _out/1 -> Output/1
  _out/2 -> Terminator/1
  Constant/1 -> _out/1

== system Simple_lib/Electronics/Forward ==
  In1 : Inport
  Bus Creator : BusCreator  Inputs=3
  Bus Selector1 : BusSelector  OutputSignals=I
  Bus Selector2 : BusSelector  OutputSignals=I,C,G
  Compare To Zero : simulink/Logic and Bit Operations/Compare To Zero  relop=<=  OutDataTypeStr=boolean
  Constant : Constant  Value=V_drop
  Divide2 : Product  Inputs=*/
  Ground{,1..3} (4 alike) : Ground
  Integrator (Discrete or Continuous) : peGeneralControl/Integrator (Discrete or Continuous)  LabelModeActiveChoice=Discrete  ExternalReset=level  LimitType=Anti-windup  B=V_drop  A=-inf  Ts=-1
  Sum : Sum  Inputs=|+-
  Switch : Switch  Criteria=u2 ~= 0
  Switch1 : Switch  Criteria=u2 ~= 0
  Weighted Sample Time : SampleTimeMath  TsampMathOp=*
  _in : $bdroot/Electronics/_in  Level=V  Flow=I
  _out : $bdroot/Electronics/_out  Tag=Electrical  Level=V  Flow=I
  Out1 : Outport
  wires:
  Integrator (Discrete or Continuous)/1 -> Sum/2
  _out/1 -> Out1/1
  Sum/1 -> _out/1
  _in/1 -> Sum/1
  In1/1 -> _in/1
  Divide2/1 -> Integrator (Discrete or Continuous)/1
  Ground/1 -> Integrator (Discrete or Continuous)/2
  Constant/1 -> Integrator (Discrete or Continuous)/3
  Switch1/1 -> _in/2
  Bus Selector1/1 -> Compare To Zero/1  "<I>"
  Switch/1 -> Divide2/2
  Bus Selector2/2 -> Switch/1, Switch/2  "<C>"
  Bus Selector2/3 -> Weighted Sample Time/1  "<G>"
  Weighted Sample Time/1 -> Switch/3
  Bus Selector2/1 -> Divide2/1  "<I>"
  _out/2 -> Bus Selector1/1, Bus Selector2/1, Switch1/3
  Compare To Zero/1 -> ?
  Bus Creator/1 -> Switch1/1
  Ground1/1 -> Bus Creator/1  "I"
  Ground2/1 -> Bus Creator/2  "G"
  Ground3/1 -> Bus Creator/3  "C"

== system Simple_lib/Electronics/Gnd ==
  Constant : Constant  Value=0
  _out : $bdroot/Electronics/_out  Tag=Electrical  Level=V  Flow=I
  Gnd : Outport
  I : Outport  Port=2
  wires:
  _out/1 -> Gnd/1
  Constant/1 -> _out/1
  _out/2 -> I/1

== system Simple_lib/Electronics/IdealSwitch ==
  s : Inport
  In2 : Inport  Port=2
  Abs : Abs
  Bus Selector1 : BusSelector  OutputSignals=I,G,C
  Compare To Zero : simulink/Logic and Bit Operations/Compare To Zero  relop===  OutDataTypeStr=boolean
  Ground : Ground
  Integrator (Discrete or Continuous) : peGeneralControl/Integrator (Discrete or Continuous)  LabelModeActiveChoice=Discrete  ExternalReset=level  LimitType=Anti-windup  B=inf  A=-inf  Ts=systemTs
  Multiply : Product  Inputs=*/
  Saturation : Saturate  UpperLimit=inf  LowerLimit=1e-12
      settings: AttributesFormatString=|
      | %<UpperLimit>
      | %<LowerLimit>
  Sum : Sum  Inputs=|+-
  Switch2 : Switch  Criteria=u2 ~= 0
  Weighted Sample Time2 : SampleTimeMath  TsampMathOp=*  weightValue=1
  _in : $bdroot/Electronics/_in  Level=V  Flow=I
  _out : $bdroot/Electronics/_out  Tag=Electrical  Level=V  Flow=I
  Out1 : Outport
  wires:
  Ground/1 -> Integrator (Discrete or Continuous)/3
  Multiply/1 -> Integrator (Discrete or Continuous)/1
  Bus Selector1/3 -> Compare To Zero/1, Switch2/3  "<C>"
  Bus Selector1/2 -> Weighted Sample Time2/1  "<G>"
  _out/2 -> Bus Selector1/1, _in/2
  Switch2/1 -> Abs/1  "C"
  Abs/1 -> Saturation/1
  Weighted Sample Time2/1 -> Switch2/1  "C"
  Compare To Zero/1 -> Switch2/2
  Bus Selector1/1 -> Multiply/1  "<I>"
  Saturation/1 -> Multiply/2
  In2/1 -> _in/1
  s/1 -> Integrator (Discrete or Continuous)/2
  _out/1 -> Out1/1
  _in/1 -> Sum/1
  Sum/1 -> _out/1
  Integrator (Discrete or Continuous)/1 -> Sum/2

== system Simple_lib/Electronics/Isrc ==
  pos : Inport
  I : Inport  Port=2
  neg : Inport  Port=3
  1/R1 : Gain  Gain=-1
  1/R2 : Gain  Gain=-1
  Bus Creator : BusCreator  Inputs=3
  Bus Creator1 : BusCreator  Inputs=3
  Ground : Ground
  Ground1 : Ground
  Ground2 : Ground
  Sum : Sum  Inputs=+|+
  _neg : $bdroot/Electronics/Isrc/_pos
      mask init:
      | initInput
      mask Display:
      | % This is a new mask on top of the base mask.
      | % Use "View base mask" link below to see the base mask.
      | %% Icon for flow in
      | % Signally design
      | %plot([0 2 2 3], [1 1 0 0])
      | %plot([1 3 2 1 0 2], [0.6 0.6 0.4 0.6 0.4 0.4])
      | %patch([1 3 2],[0.6 0.6 0.4])
      | %plot([0 1 1], [1 1 0.6])
      | %plot([1 1 0], [0.4 -1 -1])
      | 
      | %color('white')
      | %plot([0 3], [2 2])
      | %plot([0 3], [-2 -2])
      | 
      | %% Bolder design
      | %patch( [0 1 -1], [0 1 1])
      | patch( [-0.1 -0.1 -1], [0.95 0 0.95])
      | patch( [0.1 0.1 1], [1 0 1])
      | plot( [0.1 1 -1 -0.1], [0 -2 -2 0]*0.5)
      | %patch( [-0.1 0.1 0.1 -0.1], [0 0 1 1], [1 1 1])
      | %patch( [-1 0.1 0.1 -1], [1 1 0.95 0.95], [1 1 1])
      | 
      | %% Size the box
      | color('white')
      | plot( [-1 1], [2 2])
      | plot( [-1 1], -[2 2])
  _pos : $bdroot/Electronics/_in  Level=V  Flow=I
      mask init:
      | initInput
      mask Display:
      | % This is a new mask on top of the base mask.
      | % Use "View base mask" link below to see the base mask.
      | %% Icon for flow in
      | % Signally design
      | %plot([0 2 2 3], [1 1 0 0])
      | %plot([1 3 2 1 0 2], [0.6 0.6 0.4 0.6 0.4 0.4])
      | %patch([1 3 2],[0.6 0.6 0.4])
      | %plot([0 1 1], [1 1 0.6])
      | %plot([1 1 0], [0.4 -1 -1])
      | 
      | %color('white')
      | %plot([0 3], [2 2])
      | %plot([0 3], [-2 -2])
      | 
      | %% Bolder design
      | %patch( [0 1 -1], [0 1 1])
      | patch( [-0.1 -0.1 -1], [0.95 0 0.95])
      | patch( [0.1 0.1 1], [1 0 1])
      | plot( [0.1 1 -1 -0.1], [0 -2 -2 0]*0.5)
      | %patch( [-0.1 0.1 0.1 -0.1], [0 0 1 1], [1 1 1])
      | %patch( [-1 0.1 0.1 -1], [1 1 0.95 0.95], [1 1 1])
      | 
      | %% Size the box
      | color('white')
      | plot( [-1 1], [2 2])
      | plot( [-1 1], -[2 2])
  V : Outport
  wires:
  1/R1/1 -> Bus Creator1/3  "I"
  Ground1/1 -> Bus Creator1/2  "C"
  Bus Creator1/1 -> _neg/2
  _neg/1 -> Sum/2
  neg/1 -> _neg/1
  Sum/1 -> V/1
  _pos/1 -> 1/R2/1
  pos/1 -> _pos/1
  Bus Creator/1 -> _pos/2
  1/R2/1 -> Sum/1
  I/1 -> 1/R1/1, Bus Creator/2  "I"
  Ground/1 -> Bus Creator/1  "C"
  Ground2/1 -> Bus Creator/3, Bus Creator1/1  "G"

== system Simple_lib/Electronics/L ==
  In1 : Inport
  In2 : Inport  Port=2
  1/R1 : Gain  Gain=1/L
  1/R5 : Gain  Gain=-1
  Bus Creator : BusCreator  Inputs=3
  Bus Creator1 : BusCreator  Inputs=3
  Constant : Constant  Value=V_0
  Ground : Ground
  Ground1 : Ground
  Ground2 : Ground
  Integrator (Discrete or Continuous) : peGeneralControl/Integrator (Discrete or Continuous)  LabelModeActiveChoice=Discrete  ExternalReset=level  LimitType=Anti-windup  B=inf  A=-inf  Ts=systemTs
  Sum : Sum  Inputs=-|+
  _in : $bdroot/Electronics/_in  Level=V  Flow=I
      mask init:
      | initInput
      mask Display:
      | % This is a new mask on top of the base mask.
      | % Use "View base mask" link below to see the base mask.
      | %% Icon for flow in
      | % Signally design
      | %plot([0 2 2 3], [1 1 0 0])
      | %plot([1 3 2 1 0 2], [0.6 0.6 0.4 0.6 0.4 0.4])
      | %patch([1 3 2],[0.6 0.6 0.4])
      | %plot([0 1 1], [1 1 0.6])
      | %plot([1 1 0], [0.4 -1 -1])
      | 
      | %color('white')
      | %plot([0 3], [2 2])
      | %plot([0 3], [-2 -2])
      | 
      | %% Bolder design
      | %patch( [0 1 -1], [0 1 1])
      | patch( [-0.1 -0.1 -1], [0.95 0 0.95])
      | patch( [0.1 0.1 1], [1 0 1])
      | plot( [0.1 1 -1 -0.1], [0 -2 -2 0]*0.5)
      | %patch( [-0.1 0.1 0.1 -0.1], [0 0 1 1], [1 1 1])
      | %patch( [-1 0.1 0.1 -1], [1 1 0.95 0.95], [1 1 1])
      | 
      | %% Size the box
      | color('white')
      | plot( [-1 1], [2 2])
      | plot( [-1 1], -[2 2])
  _out : $bdroot/Electronics/_in  Level=V  Flow=I
      mask init:
      | initInput
      mask Display:
      | % This is a new mask on top of the base mask.
      | % Use "View base mask" link below to see the base mask.
      | %% Icon for flow in
      | % Signally design
      | %plot([0 2 2 3], [1 1 0 0])
      | %plot([1 3 2 1 0 2], [0.6 0.6 0.4 0.6 0.4 0.4])
      | %patch([1 3 2],[0.6 0.6 0.4])
      | %plot([0 1 1], [1 1 0.6])
      | %plot([1 1 0], [0.4 -1 -1])
      | 
      | %color('white')
      | %plot([0 3], [2 2])
      | %plot([0 3], [-2 -2])
      | 
      | %% Bolder design
      | %patch( [0 1 -1], [0 1 1])
      | patch( [-0.1 -0.1 -1], [0.95 0 0.95])
      | patch( [0.1 0.1 1], [1 0 1])
      | plot( [0.1 1 -1 -0.1], [0 -2 -2 0]*0.5)
      | %patch( [-0.1 0.1 0.1 -0.1], [0 0 1 1], [1 1 1])
      | %patch( [-1 0.1 0.1 -1], [1 1 0.95 0.95], [1 1 1])
      | 
      | %% Size the box
      | color('white')
      | plot( [-1 1], [2 2])
      | plot( [-1 1], -[2 2])
  wires:
  Bus Creator1/1 -> _in/2
  Bus Creator/1 -> _out/2
  In2/1 -> _out/1
  Integrator (Discrete or Continuous)/1 -> 1/R1/1  "I"
  1/R5/1 -> Bus Creator1/1  "I"
  In1/1 -> _in/1
  _in/1 -> Sum/1
  _out/1 -> Sum/2
  Ground/1 -> Bus Creator/2, Bus Creator1/2  "C"
  Ground1/1 -> Integrator (Discrete or Continuous)/1
  Constant/1 -> Integrator (Discrete or Continuous)/3
  Sum/1 -> Integrator (Discrete or Continuous)/2
  1/R1/1 -> 1/R5/1, Bus Creator/1  "I"
  Ground2/1 -> Bus Creator1/3, Bus Creator/3  "G"

== system Simple_lib/Electronics/L0 ==
  In1 : Inport
  In2 : Inport  Port=2
  1/R5 : Gain  Gain=-1
  Constant : Constant  Value=0
  Constant1 : Constant  Value=0
  Discrete-Time Integrator1 : DiscreteIntegrator  gainval=1/L  SampleTime=Ts  ICPrevOutput=DiscIntNeverNeededParam  ICPrevScaledInput=DiscIntNeverNeededParam
  Real-Imag to Complex : RealImagToComplex
  Real-Imag to Complex1 : RealImagToComplex
  Sum : Sum  Inputs=-|+
  _1 : $bdroot/Electronics/In
      mask init:
      | initInput
      mask Display:
      | % This is a new mask on top of the base mask.
      | % Use "View base mask" link below to see the base mask.
      | %% Icon for flow in
      | % Signally design
      | %plot([0 2 2 3], [1 1 0 0])
      | %plot([1 3 2 1 0 2], [0.6 0.6 0.4 0.6 0.4 0.4])
      | %patch([1 3 2],[0.6 0.6 0.4])
      | %plot([0 1 1], [1 1 0.6])
      | %plot([1 1 0], [0.4 -1 -1])
      | 
      | %color('white')
      | %plot([0 3], [2 2])
      | %plot([0 3], [-2 -2])
      | 
      | %% Bolder design
      | %patch( [0 1 -1], [0 1 1])
      | patch( [-0.1 -0.1 -1], [0.95 0 0.95])
      | patch( [0.1 0.1 1], [1 0 1])
      | plot( [0.1 1 -1 -0.1], [0 -2 -2 0]*0.5)
      | %patch( [-0.1 0.1 0.1 -0.1], [0 0 1 1], [1 1 1])
      | %patch( [-1 0.1 0.1 -1], [1 1 0.95 0.95], [1 1 1])
      | 
      | %% Size the box
      | color('white')
      | plot( [-1 1], [2 2])
      | plot( [-1 1], -[2 2])
  _2 : $bdroot/Electronics/In
      mask init:
      | initInput
      mask Display:
      | % This is a new mask on top of the base mask.
      | % Use "View base mask" link below to see the base mask.
      | %% Icon for flow in
      | % Signally design
      | %plot([0 2 2 3], [1 1 0 0])
      | %plot([1 3 2 1 0 2], [0.6 0.6 0.4 0.6 0.4 0.4])
      | %patch([1 3 2],[0.6 0.6 0.4])
      | %plot([0 1 1], [1 1 0.6])
      | %plot([1 1 0], [0.4 -1 -1])
      | 
      | %color('white')
      | %plot([0 3], [2 2])
      | %plot([0 3], [-2 -2])
      | 
      | %% Bolder design
      | %patch( [0 1 -1], [0 1 1])
      | patch( [-0.1 -0.1 -1], [0.95 0 0.95])
      | patch( [0.1 0.1 1], [1 0 1])
      | plot( [0.1 1 -1 -0.1], [0 -2 -2 0]*0.5)
      | %patch( [-0.1 0.1 0.1 -0.1], [0 0 1 1], [1 1 1])
      | %patch( [-1 0.1 0.1 -1], [1 1 0.95 0.95], [1 1 1])
      | 
      | %% Size the box
      | color('white')
      | plot( [-1 1], [2 2])
      | plot( [-1 1], -[2 2])
  wires:
  Real-Imag to Complex/1 -> _1/2
  Constant1/1 -> Real-Imag to Complex1/1
  Real-Imag to Complex1/1 -> _2/2
  Constant/1 -> Real-Imag to Complex/1
  In2/1 -> _2/1
  Discrete-Time Integrator1/1 -> 1/R5/1, Real-Imag to Complex1/2
  1/R5/1 -> Real-Imag to Complex/2
  In1/1 -> _1/1
  _1/1 -> Sum/1
  Sum/1 -> Discrete-Time Integrator1/1
  _2/1 -> Sum/2

== system Simple_lib/Electronics/L1 ==
  note: $\Phi \text{ is in Weber = Volt seconds} }$
  V_in : Inport
  at : $bdroot/Electronics/L  L=L  V_0=1e3
      settings: AttributesFormatString=|
      | %<L> H
      | %<R> Ohm
  from : $bdroot/Electronics/TP  V_0=0  slew_rate=100.0
  V_out : Outport
  wires:
  V_in/1 -> at/1
  from/1 -> at/2, V_out/1
